simulink model "SMD_SysRes"  (R2015a)
settings: Solver=ode45  StartTime=0.0  StopTime=10.0  RelTol=1e-3
settings Model: Creator=Kunal  LastModifiedBy=Kunal

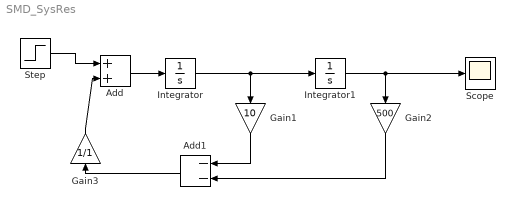
== system SMD_SysRes ==
  Add : Sum
  Add1 : Sum  Inputs=--
  Gain1 : Gain  Gain=10
  Gain2 : Gain  Gain=500
  Gain3 : Gain  Gain=1/1
  Integrator : Integrator
  Integrator1 : Integrator
  Scope : Scope
  Step : Step  SampleTime=0
  wires:
  Integrator/1 -> Integrator1/1, Gain1/1
  Integrator1/1 -> Scope/1, Gain2/1
  Gain1/1 -> Add1/1
  Add1/1 -> Gain3/1
  Gain3/1 -> Add/2
  Gain2/1 -> Add1/2
  Add/1 -> Integrator/1
  Step/1 -> Add/1
